simulink model "main_simulator"  (R2021b)
settings: Solver=ode45  StartTime=0.0  StopTime=250  RelTol=1e-3
values from neighbouring files (symbols this model uses):
  a_w = -0.00385    [ParamSetup.m]
  B_r_BP = [0; 0; -1.2]    [ParamSetup.m]    (also in param_set.m = [0; 0; -1.0])
  B_r_BW = [0; 0; 0.1]    [ParamSetup.m]    (also in param_set.m)
  C_BP = eye(3)    [ParamSetup.m]    (also in param_set.m)
  C_BW = eye(3)    [ParamSetup.m]    (also in param_set.m)
  c_Dpd = 3.2    [ParamSetup.m]    (also in param_set.m = 0.5)
  c_Yb = 0.23    [ParamSetup.m]    (also in param_set.m)
  cD = [c_D0; c_Da2; c_Dds]    [ParamSetup.m]    (also in param_set.m = [c_D0; c_DA2; c_DBs; c_DBa])
  cL = [c_L0; c_La; c_Lds]    [ParamSetup.m]    (also in param_set.m = [c_L0; c_LA; c_LBs; c_LBa])
  cM = [c_lp; c_lda; c_m0; c_ma; c_mq; c_nr; c_nda]    [ParamSetup.m]    (also in param_set.m = [c_lp; c_lBa; c_m0; c_mA; c_mq; c_nr; c_nBa])
  F = 0.0555 * (1+8*a_bar^2)*t^2*b^3    [ImIiCompute.m]    (also in param_set.m)
  gravity_acc = + 9.81    (= 9.81)    [ParamSetup.m]    (also in param_set.m)
  heights = linspace(1e-6, 350, wind_pf_size)    [Casadi_guidance.m]    (also in ParamSetup.m = linspace(1e-6, height_lim, wind_pf_size))
  Ii = diag([D, E, F])    [ImIiCompute.m]    (also in param_set.m)
  Im = diag([A, B, C])    [ImIiCompute.m]    (also in param_set.m)
  parafoil_ref_area = 1.5    [ParamSetup.m]    (also in param_set.m)
  parafoil_ref_length = 0.80    (= 0.8)    [ParamSetup.m]    (also in param_set.m)
  parafoil_ref_span = 1.88    [ParamSetup.m]    (also in param_set.m)
  psi_dot_max = 0.2187    [MPC.m]    (also in MPC_2d_path_following_func.m; MPC_2d_path_following_ground_func.m; MPC_3d_path_following.m; MPC_3d_path_following_func.m)
  r = 1000    [MPC.m]
  S_pd = 0.06    [ParamSetup.m]    (also in param_set.m)
  system_mass = 2.2    [ParamSetup.m]    (also in param_set.m)
  wind_profile_hat = GetWindProfile(heights)    [Casadi_guidance.m]    (also in ParamSetup.m)
  xy_dot = 4.59    [MPC.m]    (also in MPC_2d_path_following_func.m; MPC_2d_path_following_ground_func.m; MPC_3d_path_following.m; MPC_3d_path_following_func.m)
  z_dot = 1.39    [MPC.m]    (also in MPC_2d_path_following_func.m; MPC_2d_path_following_ground_func.m; MPC_3d_path_following.m; MPC_3d_path_following_func.m)
undefined symbols (not defined in the file or in its folder): aeroF_est_noise_var, Delta_s, diag_sigma_zeta, Light, MIL, normalize_const, psi_desire, sampling_T, time_horizon_N, wind_est_dyn_var, wind_est_noise_var, xi
libraries: aerolibwind2 x3, simulink x2, sharedtransform x1, shared6dof x1, sensorinslib x1, aerolibatmos2 x1, uavutilslib x1, commchan3 x1, matrix_library x1
settings Model: Creator=zhongyuliang  LastModifiedBy=zhongyuliang

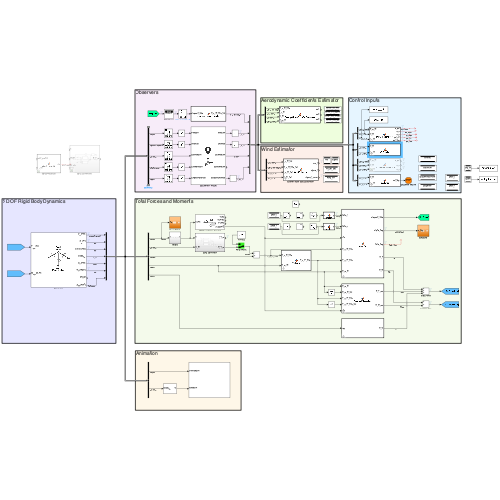
[thumbnail: Simulink's stored preview of the top-level diagram]
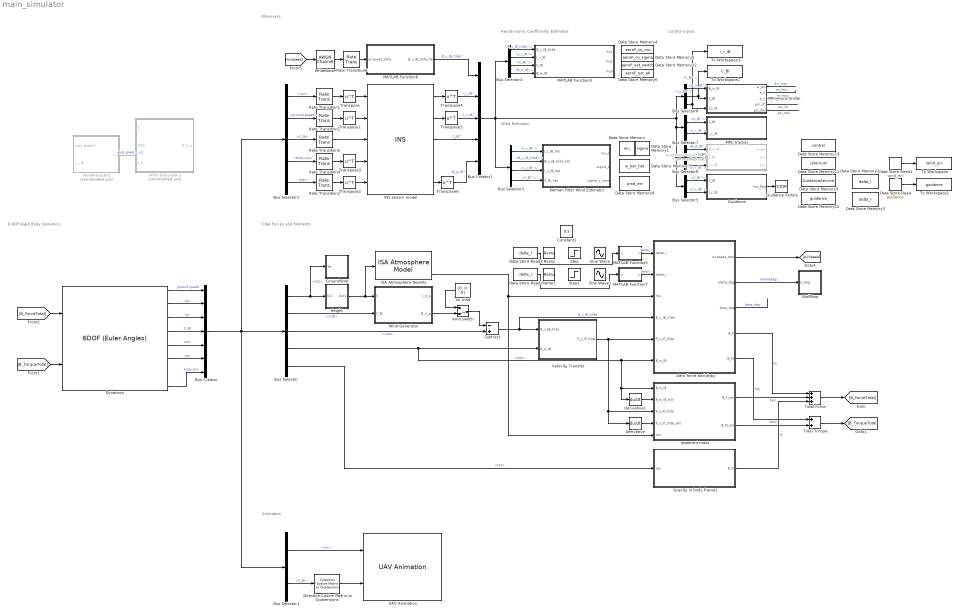
== system main_simulator ==
  note: Total Forces and Moments
  note: Animation
  note: 6 DOF Rigid Body Dynamics
  note: Observers
  note: Wind Estimator
  note: Aerodynamic Coefficients Estimator
  note: Control Inputs
  Aero force and drag : MATLAB Function  TreatAsAtomicUnit=on  mask{cL=cL, cD=cD, cYb=c_Yb, cM=cM, b=parafoil_ref_span, c=parafoil_ref_length, ref_area=parafoil_ref_area, B_r_BP=B_r_BP, C_BP=C_BP, S_pd=S_pd, c_Dpd=c_Dpd, B_r_BW=B_r_BW, C_BW=C_BW}
      mask prompts: cL "lift force coefficients"; cD "drag force coefficients"; cYb "side force coefficients"; cM "moment coefficients"; b "parafoil_ref_span"; c "parafoil_ref_length"; ref_area "parafoil_ref_area"; B_r_BP "origin deviation B_r_BP"; C_BP "rotation matrix C_BP"; S_pd "payload ref area"; c_Dpd "payload drag coefficient"; B_r_BW "origin deviation B_r_BW"; C_BW "rotation matrix C_BW"
  Bus Creator : BusCreator  Inputs=7
  Bus Creator1 : BusCreator  Inputs=5
  Bus Selector : BusSelector  OutputSignals=xyz,C_BI,uvw,pqr,rpy
  Bus Selector1 : BusSelector  OutputSignals=xyz,C_BI
  Bus Selector2 : BusSelector  OutputSignals=xyz,ground speed,C_BI,body acc,pqr
  Bus Selector3 : BusSelector  OutputSignals=I_r_IB^,B_v_IB_tilde^,I_v_IB^,C_BI^
  Bus Selector4 : BusSelector  OutputSignals=B_v_IB_tilde^,I_r_IB^,C_BI^,B_w_IB^
  Bus Selector5 : BusSelector  OutputSignals=C_BI^,I_r_IB^
  Bus Selector6 : BusSelector  OutputSignals=B_w_IB^,C_BI^,I_r_IB^
  Bus Selector7 : BusSelector  OutputSignals=C_BI^,I_r_IB^
  Bus Selector8 : BusSelector  OutputSignals=B_w_IB^,C_BI^,I_r_IB^
  Constant1 : Constant  Value=0.5
  Data Store Memory : DataStoreMemory  DataStoreName=mu  ReadBeforeWriteMsg=warning  WriteAfterWriteMsg=warning  WriteAfterReadMsg=warning  InitialValue=mu0  VectorParams1D=off  ShowAdditionalParam=off  OutDataTypeStr=double
  Data Store Memory1 : DataStoreMemory  DataStoreName=sigma  ReadBeforeWriteMsg=warning  WriteAfterWriteMsg=warning  WriteAfterReadMsg=warning  InitialValue=sigma0  VectorParams1D=off  ShowAdditionalParam=off  OutDataTypeStr=double
  Data Store Memory10 : DataStoreMemory  DataStoreName=guidance  ReadBeforeWriteMsg=warning  WriteAfterWriteMsg=warning  WriteAfterReadMsg=warning  InitialValue=zeros(4,2000)  ShowAdditionalParam=off  OutDataTypeStr=double
  Data Store Memory11 : DataStoreMemory  DataStoreName=colornum  ReadBeforeWriteMsg=warning  WriteAfterWriteMsg=warning  WriteAfterReadMsg=warning  InitialValue=randi([1,11],1)  ShowAdditionalParam=off  OutDataTypeStr=double
  Data Store Memory12 : DataStoreMemory  DataStoreName=aeroF_est_switch  ReadBeforeWriteMsg=warning  WriteAfterWriteMsg=warning  WriteAfterReadMsg=warning  InitialValue=[0,0]  VectorParams1D=off  ShowAdditionalParam=off  OutDataTypeStr=double
  Data Store Memory13 : DataStoreMemory  DataStoreName=control  ReadBeforeWriteMsg=warning  WriteAfterWriteMsg=warning  WriteAfterReadMsg=warning  InitialValue=control0  ShowAdditionalParam=off  OutDataTypeStr=double
  Data Store Memory2 : DataStoreMemory  DataStoreName=delta_l  ReadBeforeWriteMsg=warning  WriteAfterWriteMsg=warning  WriteAfterReadMsg=warning  InitialValue=0.5  ShowAdditionalParam=off  OutDataTypeStr=double
  Data Store Memory3 : DataStoreMemory  DataStoreName=delta_r  ReadBeforeWriteMsg=warning  WriteAfterWriteMsg=warning  WriteAfterReadMsg=warning  InitialValue=0.5  ShowAdditionalParam=off  OutDataTypeStr=double
  Data Store Memory4 : DataStoreMemory  DataStoreName=aeroF_co_mu  ReadBeforeWriteMsg=warning  WriteAfterWriteMsg=warning  WriteAfterReadMsg=warning  InitialValue=aeroF_co_mu0  VectorParams1D=off  ShowAdditionalParam=off  OutDataTypeStr=double
  Data Store Memory5 : DataStoreMemory  DataStoreName=aeroF_co_sigma  ReadBeforeWriteMsg=warning  WriteAfterWriteMsg=warning  WriteAfterReadMsg=warning  InitialValue=aeroF_co_sigma0  VectorParams1D=off  ShowAdditionalParam=off  OutDataTypeStr=double
  Data Store Memory6 : DataStoreMemory  DataStoreName=aeroF_est_ab  ReadBeforeWriteMsg=warning  WriteAfterWriteMsg=warning  WriteAfterReadMsg=warning  InitialValue=[0, 0, 0; 0, 0, 0]  VectorParams1D=off  ShowAdditionalParam=off  OutDataTypeStr=double
  Data Store Memory7 : DataStoreMemory  DataStoreName=w_bar_hat  ReadBeforeWriteMsg=warning  WriteAfterWriteMsg=warning  WriteAfterReadMsg=warning  InitialValue=w_bar_hat0  VectorParams1D=off  ShowAdditionalParam=off  OutDataTypeStr=double
  Data Store Memory8 : DataStoreMemory  DataStoreName=wind_err  ReadBeforeWriteMsg=warning  WriteAfterWriteMsg=warning  WriteAfterReadMsg=warning  InitialValue=wind_err0  VectorParams1D=off  ShowAdditionalParam=off  OutDataTypeStr=double
  Data Store Memory9 : DataStoreMemory  DataStoreName=GuidanceService  ReadBeforeWriteMsg=warning  WriteAfterWriteMsg=warning  WriteAfterReadMsg=warning  InitialValue=1  ShowAdditionalParam=off  OutDataTypeStr=double
  Data Store Read : DataStoreRead  DataStoreName=guidance  IndexOptions=Index vector (dialog)  Indices=1  OutputSizes=1
  Data Store Read1 : DataStoreRead  DataStoreName=wind_err  IndexOptions=Index vector (dialog)  Indices=1  OutputSizes=1
  Data Store Read2 : DataStoreRead  DataStoreName=delta_l  IndexOptions=Index vector (dialog)  Indices=1  OutputSizes=1
  Data Store Read3 : DataStoreRead  DataStoreName=delta_r  IndexOptions=Index vector (dialog)  Indices=1  OutputSizes=1
  Derivative : Derivative
  Derivative1 : Derivative
  Direction Cosine Matrix to Quaternions : sharedtransform/Direction Cosine Matrix  to Quaternions  aMode=0  action=None  tolerance=eps(2)
      settings: SourceProductBaseCode=AE,PW,DR,MT,UV,VE
  Dynamics : shared6dof/6DOF (Euler Angles)  units=Metric (MKS)  mtype=Fixed  rep=Euler Angles  xme_0=init_pos_in_inertial_frame  Vm_0=init_uvw  eul_0=init_rpy  pm_0=init_pqr  mass_0=system_mass  mass_e=0.5  mass_f=2.0  inertia=system_inertia  inertia_e=eye(3)  inertia_f=2*eye(3)  k_quat=1.0  vre_flag=on  abi_flag=off  aMode=0  xme_statename=''  Vm_statename=''  eul_statename=''  quat_statename=''  pm_statename=''  mass_statename=''
      settings: SourceProductBaseCode=AE,PW,DR,MT,UV,VE
  Gravity in body frame1 : MATLAB Function  ClipboardFcn="m = load(\"params.mat\",\"system_mass\")"  TreatAsAtomicUnit=on  mask{m=system_mass, g=gravity_acc}
      mask prompts: m "system_mass"; g "gravity_acc"
  GroundStop : Subsystem
  Guidance : MATLAB Function  TreatAsAtomicUnit=on  SystemSampleTime=25  mask{heights=heights, Delta_s=Delta_s, z_dot=z_dot, xy_dot=xy_dot, psi_dot_max=psi_dot_max, psi_d=psi_desire}
      mask prompts: Delta_s "wind pos deviation"; z_dot "descending rate no wind"; xy_dot "horizontal vel no wind"; psi_dot_max "max turning rate no wind"; psi_d "desired landing pose"
  Guidance Failure : Stop
  GuidancePDcontroller : MATLAB Function  Commented=on  TreatAsAtomicUnit=on
  Height : Subsystem
  INS sensor model : sensorinslib/INS  MountingLocation=[0 0 0]  RollAccuracy=row_pitch_accu  PitchAccuracy=row_pitch_accu  YawAccuracy=yaw_accu  PositionAccuracy=pos_accu  VelocityAccuracy=vel_accu  UseAccelAndAngVel=on  AccelerationAccuracy=acc_accu  AngularVelocityAccuracy=angVel_accu  TimeInput=off  PositionErrorFactor=[0 0 0]  SeedDouble=67  SimulateUsing=Interpreted execution
      settings: SourceProductBaseCode=DR,TF,NV,UV
  ISA Atmosphere Density : aerolibatmos2/ISA Atmosphere Model  custom=off  g=9.80665  gamma=1.4  R=287.0531  L=0.0065  h_trop=11000  h_strat=20000  rho0=1.225  P0=101325  T0=288.15  h0=0
  Kalman Filter Wind Estimator : MATLAB Function  TreatAsAtomicUnit=on  mask{Q=wind_est_dyn_var, R=wind_est_noise_var, heights=heights, wind_profile_hat=wind_profile_hat, C=normalize_const}
      mask prompts: Q "wind_est_dyn_var"; R "wind_est_noise_var"; wind_profile_hat "forcast wind profile"; C "normalize_const"
  MATLAB Function3 : MATLAB Function  TreatAsAtomicUnit=on  mask{m=system_mass, g=gravity_acc, C_BP=C_BP, C_BW=C_BW, ref_area=parafoil_ref_area, S_pd=S_pd, R=aeroF_est_noise_var}
      mask prompts: m "system_mass"; g "gravity_acc"; C_BP "rotation matrix C_BP"; C_BW "rotation matrix C_BW"; ref_area "parafoil_ref_area"; S_pd "payload_ref_area"; R "aeroF_est_noise_var"
  MATLAB Function5 : MATLAB Function  TreatAsAtomicUnit=on
  MATLAB Function6 : MATLAB Function  TreatAsAtomicUnit=on
  MATLAB Function7 : MATLAB Function  TreatAsAtomicUnit=on
  MPC tracker : MATLAB Function  TreatAsAtomicUnit=on  SystemSampleTime=2.38  mask{xy_dot=xy_dot, z_dot=z_dot, psi_dot_max=psi_dot_max, N=time_horizon_N}
      mask prompts: N "MPC time horizon"
  MPC_PDcontroller : MATLAB Function  TreatAsAtomicUnit=on
  Ramp : simulink/Sources/Ramp  slope=0.03  start=10  InitialOutput=0.5
  Ramp1 : simulink/Sources/Ramp  slope=-0.03  start=10  InitialOutput=0.5
  Rate Transition{1..6} (6 alike) : RateTransition  OutPortSampleTime=sampling_T
  Sine Wave : Sin  Amplitude=0.5  Bias=0.5  SampleTime=0
  Sine Wave1 : Sin  Amplitude=0.5  Bias=0.5  SampleTime=0
  StallStop : Subsystem
  Step : Step  Time=20  SampleTime=0
  Step1 : Step  Time=20  SampleTime=0
  Subtract : Sum  Inputs=-+
  To Workspace : ToWorkspace  VariableName=wind_err  SaveFormat=Structure With Time  SampleTime=-1
  To Workspace1 : ToWorkspace  VariableName=guidance  SaveFormat=Structure With Time  SampleTime=-1
  To Workspace2 : ToWorkspace  VariableName=C_BI  SaveFormat=Structure With Time  SampleTime=-1
  To Workspace3 : ToWorkspace  VariableName=I_r_IB  SaveFormat=Structure With Time  SampleTime=-1
  Total Force : Sum  Inputs=+++
  Total Torque : Sum
  Transpose{,1..6} (7 alike) : Math  Operator=transpose  SaturateOnIntegerOverflow=on
  UAV Animation : uavutilslib/UAV Animation  UAVType=FixedWing  UAVSize=40  InertialZDirection=Down  SampleTime=-1
      settings: SourceProductBaseCode=UV
  Velovity Transfer : MATLAB Function  TreatAsAtomicUnit=on  mask{B_r_BP=B_r_BP, C_BP=C_BP}
  WhiteNoise : commchan3/AWGN Channel  InputProcessing=Columns as channels (frame based)  seed=67  noiseMode=Variance from mask  EbNodB=10  EsNodB=10  SNRdB=100  bitsPerSym=1  Ps=1  Tsym=1  variance=airspeed_var
  Wind Generator : Subsystem
  Wind Generator1 : Subsystem  Commented=on
  WindPredictViz : MATLAB Function  Commented=on  TreatAsAtomicUnit=on  SystemSampleTime=sampling_T
  apparent mass : MATLAB Function  TreatAsAtomicUnit=on  mask{Im=Im, Ii=Ii, B_r_BP=B_r_BP, C_BP=C_BP}
      mask prompts: Im "apparent mass / air density"; Ii "apparent inertia / air density"; B_r_BP "origin deviation B_r_BP"; C_BP "rotation matrix C_BP"
  no wind : Constant  Value=[0; 0; 0]
  wind switch : ManualSwitch  CurrentSetting=0
  wires:
  Bus Selector/3 -> Subtract/2  "<uvw>"
  Height/1(Out1) -> Wind Generator/1(h), ISA Atmosphere Density/1
  Subtract/1 -> Velovity Transfer/1(B_v_IB_tilde), Aero force and drag/4(B_v_IB_tilde)  "B_v_IB_tilde"
  Velovity Transfer/1(P_v_IP_tilde) -> Aero force and drag/5(P_v_IP_tilde), apparent mass/3(P_v_IP_tilde), Derivative/1
  ISA Atmosphere Density/4 -> apparent mass/5(rho), Aero force and drag/3(rho)
  Derivative/1 -> apparent mass/4(P_v_IP_tilde_dot)
  Bus Selector/5 -> Gravity in body frame1/1(rpy)  "<rpy>"
  [B_ForceTotal] -> Dynamics/1
  [B_TorqueTotal] -> Dynamics/2
  Derivative1/1 -> apparent mass/2(B_w_IB_dot)
  Bus Selector/1 -> Height/1(In1), GroundStop/1(Xe)  "<xyz>"
  Direction Cosine Matrix to Quaternions/1 -> UAV Animation/2
  Bus Selector/4 -> Velovity Transfer/2(B_w_IB), Aero force and drag/6(B_w_IB), apparent mass/1(B_w_IB), Derivative1/1  "<pqr>"
  Dynamics/1 -> Bus Creator/1  "ground speed"
  Dynamics/2 -> Bus Creator/2  "xyz"
  Dynamics/3 -> Bus Creator/3  "rpy"
  Dynamics/4 -> Bus Creator/4  "C_BI"
  Dynamics/5 -> Bus Creator/5  "uvw"
  Dynamics/6 -> Bus Creator/6  "pqr"
  Dynamics/8 -> Bus Creator/7  "body acc"
  Bus Creator/1 -> Bus Selector/1, Bus Selector1/1, Bus Selector2/1
  Bus Selector1/1 -> UAV Animation/1  "<xyz>"
  Bus Selector1/2 -> Direction Cosine Matrix to Quaternions/1  "<C_BI>"
  Bus Selector/2 -> Wind Generator/2(C_BI)  "<C_BI>"
  MATLAB Function5/1(y) -> Aero force and drag/1(delta_l)  "delta_l"
  MATLAB Function7/1(y) -> Aero force and drag/2(delta_r)  "delta_r"
  no wind/1 -> wind switch/1
  Wind Generator/2(B_V_w) -> wind switch/2
  wind switch/1 -> Subtract/1
  Aero force and drag/1(airspeed_data) -> [AirSpeed]
  Aero force and drag/5(B_M) -> Total Torque/1  "Ma"
  Gravity in body frame1/1(B_G) -> Total Force/3  "G"
  Total Torque/1 -> [B_TorqueTotal]
  Total Force/1 -> [B_ForceTotal]
  Aero force and drag/4(B_F) -> Total Force/1  "Fa"
  apparent mass/2(B_M_am) -> Total Torque/2  "Mam"
  Aero force and drag/2(alpha_deg) -> StallStop/1(a_deg)  "alpha[deg]"
  Bus Selector2/4 -> Rate Transition4/1  "<body acc>"
  Bus Selector3/2 -> Kalman Filter Wind Estimator/2(B_v_IB_tilde_hat)  "<B_v_IB_tilde^>"
  Bus Selector3/1 -> Kalman Filter Wind Estimator/1(I_r_IB_hat)  "<I_r_IB^>"
  Rate Transition2/1 -> Transpose1/1
  MATLAB Function6/1(B_v_IB_tilde_hat) -> Bus Creator1/1  "B_v_IB_tilde^"
  Bus Selector4/4 -> MATLAB Function3/4(B_w_IB)  "<B_w_IB^>"
  Bus Selector3/4 -> Kalman Filter Wind Estimator/4(C_BI_hat)  "<C_BI^>"
  Bus Selector6/1 -> GuidancePDcontroller/1(B_w_IB)  "<B_w_IB^>"
  WhiteNoise/1 -> Rate Transition6/1
  INS sensor model/3 -> Bus Creator1/4  "C_BI^"
  Bus Selector5/1 -> Guidance/1(C_BI)  "<C_BI^>"
  Transpose/1 -> INS sensor model/1
  Rate Transition1/1 -> Transpose/1
  Rate Transition3/1 -> Transpose2/1
  Transpose3/1 -> INS sensor model/4
  [AirSpeed] -> WhiteNoise/1
  Bus Selector3/3 -> Kalman Filter Wind Estimator/3(I_v_IB_hat)  "<I_v_IB^>"
  Transpose5/1 -> Bus Creator1/3  "I_v_IB^"
  Rate Transition6/1 -> MATLAB Function6/1(airspeed_data)
  INS sensor model/5 -> Transpose6/1
  INS sensor model/1 -> Transpose4/1
  Rate Transition5/1 -> INS sensor model/3
  Bus Selector2/3 -> Rate Transition5/1  "<C_BI>"
  Guidance/1(not_flag) -> Guidance Failure/1
  Transpose2/1 -> INS sensor model/5
  Bus Selector2/1 -> Rate Transition1/1  "<xyz>"
  Bus Selector2/2 -> Rate Transition2/1  "<ground speed>"
  Bus Selector2/5 -> Rate Transition3/1  "<pqr>"
  Transpose1/1 -> INS sensor model/2
  INS sensor model/2 -> Transpose5/1
  Bus Selector6/3 -> GuidancePDcontroller/3(I_r_IB)  "<I_r_IB^>"
  Transpose6/1 -> Bus Creator1/5  "B_w_IB^"
  Bus Selector6/2 -> GuidancePDcontroller/2(C_BI)  "<C_BI^>"
  Transpose4/1 -> Bus Creator1/2  "I_r_IB^"
  Bus Selector5/2 -> Guidance/2(I_r_IB)  "<I_r_IB^>"
  Rate Transition4/1 -> Transpose3/1
  Bus Selector4/2 -> MATLAB Function3/2(I_r_IB)  "<I_r_IB^>"
  Bus Selector4/1 -> MATLAB Function3/1(B_v_IB_tilde)  "<B_v_IB_tilde^>"
  Bus Selector4/3 -> MATLAB Function3/3(C_BI)  "<C_BI^>"
  WindPredictViz/1(viz) -> ?  "wind_predict_viz"
  apparent mass/1(B_F_am) -> Total Force/2  "Fam"
  Aero force and drag/3(beta_deg) -> ?  "beta_deg"
  Data Store Read2/1 -> MATLAB Function5/1(u)
  Data Store Read3/1 -> MATLAB Function7/1(u)
  Data Store Read/1 -> To Workspace1/1
  Data Store Read1/1 -> To Workspace/1
  Bus Selector7/1 -> MPC tracker/1(C_BI)  "<C_BI^>"
  Bus Selector7/2 -> MPC tracker/2(I_r_IB)  "<I_r_IB^>"
  Bus Creator1/1 -> Bus Selector4/1, Bus Selector3/1, Bus Selector8/1, Bus Selector5/1, Bus Selector6/1, Bus Selector7/1
  Bus Selector8/1 -> MPC_PDcontroller/1(B_w_IB)  "<B_w_IB^>"
  Bus Selector8/2 -> To Workspace2/1, MPC_PDcontroller/2(C_BI)  "<C_BI^>"
  MPC_PDcontroller/1(e_psi) -> ?  "err_mpc"
  Bus Selector8/3 -> To Workspace3/1, MPC_PDcontroller/3(I_r_IB)  "<I_r_IB^>"
  MPC_PDcontroller/2(e_x) -> ?  "ex_mpc"
  MPC_PDcontroller/3(e_y) -> ?  "ey_mpc"
  MPC_PDcontroller/4(psi_ctl) -> ?  "psi_ctl"
  MPC_PDcontroller/5(psi_des) -> ?  "psi_des"

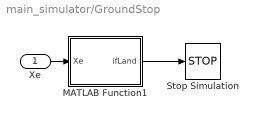
== system main_simulator/GroundStop ==
  Xe : Inport
  MATLAB Function1 : MATLAB Function  TreatAsAtomicUnit=on
  Stop Simulation : Stop
  wires:
  Xe/1 -> MATLAB Function1/1(Xe)
  MATLAB Function1/1(ifLand) -> Stop Simulation/1

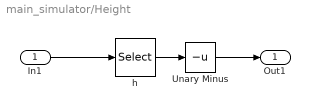
== system main_simulator/Height ==
  In1 : Inport
  Unary Minus : UnaryMinus
  h : Selector  InputPortWidth=3  IndexOptions=Index vector (dialog)  Indices=3  OutputSizes=1
  Out1 : Outport
  wires:
  Unary Minus/1 -> Out1/1
  In1/1 -> h/1
  h/1 -> Unary Minus/1

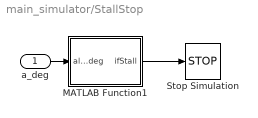
== system main_simulator/StallStop ==
  a_deg : Inport
  MATLAB Function1 : MATLAB Function  TreatAsAtomicUnit=on
  Stop Simulation : Stop
  wires:
  a_deg/1 -> MATLAB Function1/1(alpha_deg)
  MATLAB Function1/1(ifStall) -> Stop Simulation/1

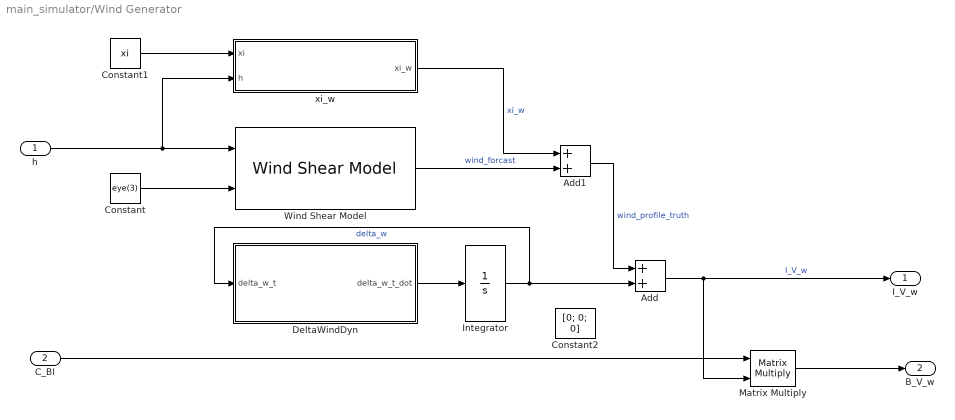
== system main_simulator/Wind Generator ==
  h : Inport
  C_BI : Inport  Port=2
  Add : Sum
  Add1 : Sum
  Constant : Constant  Value=eye(3)
  Constant1 : Constant  Value=xi
  Constant2 : Constant  Value=[0; 0; 0]
  DeltaWindDyn : MATLAB Function  TreatAsAtomicUnit=on  SystemSampleTime=0.2  mask{a_w=a_w, diag_sigma_zeta=diag_sigma_zeta}
  Integrator : Integrator
  Matrix Multiply : Product  Multiplication=Matrix(*)
  Wind Shear Model : aerolibwind2/Wind Shear Model  units=Metric (MKS)  phase=Category C - Terminal Flight Phase  W_20=vel_at6m  Wdeg=theta
  xi_w : MATLAB Function  TreatAsAtomicUnit=on
  I_V_w : Outport
  B_V_w : Outport  Port=2
  wires:
  DeltaWindDyn/1(delta_w_t_dot) -> Integrator/1
  Wind Shear Model/1 -> Add1/2  "wind_forcast"
  Add/1 -> I_V_w/1, Matrix Multiply/2  "I_V_w"
  h/1 -> xi_w/2(h), Wind Shear Model/1
  Integrator/1 -> Add/2, DeltaWindDyn/1(delta_w_t)  "delta_w"
  C_BI/1 -> Matrix Multiply/1
  Matrix Multiply/1 -> B_V_w/1
  Constant/1 -> Wind Shear Model/2
  Constant1/1 -> xi_w/1(xi)
  xi_w/1(xi_w) -> Add1/1  "xi_w"
  Add1/1 -> Add/1  "wind_profile_truth"

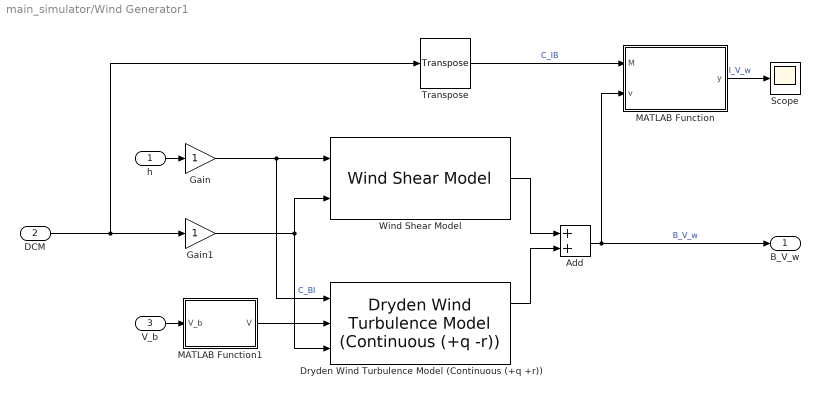
== system main_simulator/Wind Generator1 ==
  h : Inport
  DCM : Inport  Port=2
  V_b : Inport  Port=3
  Add : Sum
  Dryden Wind Turbulence Model (Continuous (+q +r)) : aerolibwind2/Dryden Wind Turbulence Model  (Continuous (+q -r))  units=Metric (MKS)  spec=MIL-F-8785C  model=Continuous Dryden (+q +r)  W20=turbulence_vel_at6m  Wdeg=turbulence_ori_at6m  TurbProb=10^-2 - Light  L_high=533.4  Wingspan=parafoil_ref_span  ts=0.1  Seed=[23341 23342 23343 23344]  T_on=on
  Gain : Gain
  Gain1 : Gain
  MATLAB Function : MATLAB Function  TreatAsAtomicUnit=on
  MATLAB Function1 : MATLAB Function  TreatAsAtomicUnit=on
  Scope : Scope
  Transpose : matrix_library/Transpose
      settings: SourceProductBaseCode=SL
  Wind Shear Model : aerolibwind2/Wind Shear Model  units=Metric (MKS)  phase=Category C - Terminal Flight Phase  W_20=laminar_wind_vel_at6m  Wdeg=laminar_wind_ori_at6m
  B_V_w : Outport
  wires:
  V_b/1 -> MATLAB Function1/1(V_b)
  DCM/1 -> Transpose/1, Gain1/1
  Dryden Wind Turbulence Model (Continuous (+q +r))/1 -> Add/2
  MATLAB Function1/1(V) -> Dryden Wind Turbulence Model (Continuous (+q +r))/2
  h/1 -> Gain/1
  Gain/1 -> Dryden Wind Turbulence Model (Continuous (+q +r))/1, Wind Shear Model/1
  Wind Shear Model/1 -> Add/1
  Gain1/1 -> Dryden Wind Turbulence Model (Continuous (+q +r))/3, Wind Shear Model/2  "C_BI"
  Add/1 -> B_V_w/1, MATLAB Function/2(v)  "B_V_w"
  MATLAB Function/1(y) -> Scope/1  "I_V_w"
  Transpose/1 -> MATLAB Function/1(M)  "C_IB"

== matlab function main_simulator/Gravity in body frame1 ==
  data: rpy input; B_G output; m parameter; g parameter
function B_G = GravityInBodyFrame(rpy, m, g)
    B_G = m*g*[-sin(rpy(2));
             sin(rpy(1))*cos(rpy(2));
             cos(rpy(1))*cos(rpy(2))];
end

== matlab function main_simulator/GroundStop/MATLAB Function1 ==
  data: Xe input; ifLand output
function ifLand = logic(Xe)

    if Xe(3) < -0.000001
        ifLand = 0;
    else
        ifLand = 1;
    end

end

== matlab function main_simulator/StallStop/MATLAB Function1 ==
  data: alpha_deg input; ifStall output
function ifStall = logic(alpha_deg)

    if alpha_deg < 45
        ifStall = 0;
    else
        ifStall = 1;
    end
%     ifStall = 0;

end

== matlab function main_simulator/Wind Generator/xi_w ==
  data: xi input; h input; xi_w output
function xi_w = fcn(xi,h)

xi_w = [xi(1) * h / 200;
        xi(2) * h / 200;
        0];
end

== matlab function main_simulator/Guidance ==
  settings: updateMethod=DISCRETE
  data: not_flag output; C_BI input; I_r_IB input; heights parameter; psi_dot_max parameter; xy_dot parameter; z_dot parameter; psi_d parameter; Delta_s parameter; guidance data_store_memory; GuidanceService data_store_memory
function not_flag = Guidance(C_BI, I_r_IB, heights, psi_dot_max, xy_dot, z_dot, psi_d, Delta_s)

    global GuidanceService;
    global guidance
    h = -I_r_IB(3);
    not_flag = false;

    
    if h<300 && h>1e-6 && GuidanceService
        disp('------Guidance------')
        Vz = z_dot;
        Dx_w = (1/Vz)*interp1(heights, Delta_s(1,:), h, 'linear','extrap');
        Dy_w = (1/Vz)*interp1(heights, Delta_s(2,:), h, 'linear','extrap');
        V0 = xy_dot / Vz;
        T = h;
        um = psi_dot_max / Vz;

        C_IB = C_BI';
        psi0 = atan2(C_IB(2,1), C_IB(1,1));
        
        init_pose = [I_r_IB(1) + Dx_w;
                     I_r_IB(2) + Dy_w;
                     psi0];
        final_pose = [0; 0; psi_d];
        
        % NLP solver
        [p_0_star, ~, flag] = fminsearch(@(P0) ComputeErr(P0, init_pose, final_pose, T, V0, um),[-1e-5,1e-5,1e-4],optimset('TolFun',1e-7,'TolX',1e-7,'MaxFunEvals',1e5,'MaxIter',1e5));
        not_flag = ~flag;
        
        % if solution found
        if flag
            t_span = linspace(0, T, 2000);
            x0 = [init_pose(1);
                  init_pose(2);
                  init_pose(3);
                  p_0_star(1);
                  p_0_star(2);
                  p_0_star(3)];
            [time, traj] = ode45(@(t,x) ODEdyn(t,x, V0, um), t_span, x0);
        
            for i = 1:2000
                guidance(:,i) = [traj(i,1) - (1/Vz)*interp1(heights, Delta_s(1,:), h - time(i),'linear','extrap'); % I_rx
                                 traj(i,2) - (1/Vz)*interp1(heights, Delta_s(2,:), h - time(i),'linear','extrap'); % I_ry
                                 h - time(i); % h, -I_rz
                                 traj(i,3)]; % psi
            end
            
            % plot
            hold on
            grid on
            xlabel('East --> y') 
            ylabel('North --> x') 
            zlabel('Height --> h')
            plot3(guidance(2,:),guidance(1,:),guidance(3,:),'k') % changed viz axis
            
        else
            disp("Warning! Guidance solver failed!")
            return % guidance fail! do not update guidance, go to teleop...
        end
        GuidanceService = 0; % task complete
    end
end

function dxdt = ODEdyn(t, x, V0, um) % x = [x, y, chi, p1, p2, p3]^T
    if(x(6) >= 2*um)
        u = -um;
    elseif(x(6) >= -2*um)
        u = -x(6)/2;
    else
        u = um;
    end
    dxdt = [V0*cos(x(3));
            V0*sin(x(3));
            u;
            0;
            0;
            x(4)*V0*sin(x(3)) - x(5)*V0*cos(x(3))];
end

function err = ComputeErr(P0, init_pose, final_pose, T, V0, um)
    t_span = linspace(0, T, 1000);
    x0 = [init_pose(1);
          init_pose(2);
          init_pose(3);
          P0(1);
          P0(2);
          P0(3)];
    [~, traj] = ode45(@(t,x) ODEdyn(t,x, V0, um), t_span, x0);
    err = sqrt((traj(end,1) - final_pose(1))^2 + (traj(end,2) - final_pose(2))^2) - 10000*((cos(traj(end,3) - final_pose(3)) -1));
end

== matlab function main_simulator/MPC tracker ==
  data: C_BI input; I_r_IB input; guidance data_store_memory; wind_err data_store_memory; z_dot parameter; xy_dot parameter; control data_store_memory; psi_dot_max parameter; N parameter; GuidanceService data_store_memory
function MPCtracker(C_BI, I_r_IB, z_dot, xy_dot, psi_dot_max, N)
    coder.extrinsic("MPC_func")

    global guidance
    global wind_err
    global control
    global GuidanceService

    % get current state
    xc = I_r_IB(1);
    yc = I_r_IB(2);
    h = -I_r_IB(3);
    C_IB = C_BI';
    psi_c = atan2(C_IB(2,1), C_IB(1,1));

    if isnan(xc) || isnan(yc) || isnan(h) || isnan(psi_c)
        disp("Warning: MPCtracker early return because of NaN current pose value")
        return
    elseif h < 1e-6
        disp("Warning: MPCtracker early return because h < 1e-6")
        return
    end

    % if guidance and wind_err received
    zero_cnt = sum(guidance==0, 'all') + sum(wind_err==0, 'all');

    if zero_cnt<3

        [~, id] = min(abs(guidance(3,:) - h*ones(1,2000)));
        x0 = guidance(1,id);
        y0 = guidance(2,id);
        dx = mean(wind_err(2,:));
        dy = mean(wind_err(3,:));
        dh = (guidance(3,1) - guidance(3,end))/(2000 - 1);
        Ts = dh / z_dot;
        init_pose = [xc - x0; yc - y0; psi_c];
        
        % Compute ref trajectory
        ref = zeros(3,N);
        ref(3,1) = guidance(4,id);
        for i = 2:N
            if id+i-1>2000
                ref(:,i) = ref(:,i-1);
            else
                ref(:,i) =  [ref(1,i-1) + Ts * xy_dot * cos(guidance(4,id+i-2));
                             ref(2,i-1) + Ts * xy_dot * sin(guidance(4,id+i-2));
                             guidance(4,id+i-1)];
            end
        end
        
        % Solve MPC problem
        flag = true;
        xs = zeros(3,N); % define output shape
        us = zeros(1,N-1); % define output shape
        P = diag([10000,10000,100]);
        Q = diag([100, 100, 10000]);
        Qn = diag([1000, 1000, 100]);
        r = 1000;
        um = psi_dot_max;
        
        if sum(isnan(init_pose),'all')>0
            disp("Warning: MPCtracker early return because of NaN initial pose value")
        elseif sum(isnan(ref),'all')>0
            disp("Warning: MPCtracker early return because of NaN reference value")
        end

        [flag, xs, ~] = MPC_func(N, init_pose, P, Q, r, Qn, ref, Ts, xy_dot, um, dx, dy);
        if flag
            if id+N-1 <= 2000
                ctl = [guidance(3,id:id+N-1);
                       xs(3,:)];
                control = ctl(:,1:size(control,2));
            else
                ctl = [guidance(3,id:2000), linspace(-dh, -dh*(N-(2000-id+1)), N-(2000-id+1));
                       xs(3,:)];
                control = ctl(:,1:size(control,2));
            end        
        else
            disp("MPC solver failed")
            GuidanceService = 1; % recall guidance, do not change control in buffer
        end
    end
end

== matlab function main_simulator/MATLAB Function5 ==
  data: u input; y output
function y = motor(u)
    if u>1
        y = 1;
    elseif u<0
        y = 0;
    else
        y = u;
    end
end

== matlab function main_simulator/MPC_PDcontroller ==
  data: B_w_IB input; C_BI input; I_r_IB input; delta_l data_store_memory; delta_r data_store_memory; guidance data_store_memory; control data_store_memory; GuidanceService data_store_memory; colornum data_store_memory; e_psi output; e_x output; e_y output; psi_ctl output; psi_des output
function [e_psi, e_x, e_y, psi_ctl, psi_des] = MPC_PDcontroller(B_w_IB, C_BI, I_r_IB)
    global delta_l
    global delta_r
    global control
    global GuidanceService
    global guidance
    global colornum
    
    % get current state
    h = -I_r_IB(3);
    C_IB = C_BI';
    x_now = I_r_IB(1);
    y_now = I_r_IB(2);
    psi_now = atan2(C_IB(2,1), C_IB(1,1));

    % plot current state
    hold on;
    colorcode = {"g","b", "c", "m", "#0072BD", "#D95319", "#EDB120", "#7E2F8E", "#77AC30", "#4DBEEE", "#A2142F"};
    states_now = [y_now,                x_now,                h;
                  y_now+1*sin(psi_now), x_now+1*cos(psi_now), h];
    plot3(states_now(:,1), states_now(:,2), states_now(:,3), 'color', colorcode{colornum});

    % default output
    e_psi = 0;
    e_x = 0;
    e_y = 0;
    psi_ctl = 0; % for debug
    psi_des = 0; % for debug
    
    if isnan(x_now) || isnan(y_now) || isnan(h) || isnan(psi_now)
        disp("Warning: MPC_PDcontroller early return because of NaN value")
        return
%     elseif h < 1e-6
%         disp("Warning: GuidancePDcontroller early return because h < 1e-6")
%         return
    end

    % get control
    zero_cnt = sum(control==0, 'all') + sum(guidance==0, 'all'); % if control and guidance received
    if zero_cnt<3
        x_des = interp1(guidance(3,:), guidance(1,:), h, 'linear','extrap'); 
        y_des = interp1(guidance(3,:), guidance(2,:), h, 'linear','extrap'); 
        psi_des = interp1(guidance(3,:), guidance(4,:), h, 'linear','extrap'); 
       
        % plot desired trajectory
        traj = [y_des,                x_des,                h;
                y_des+1*sin(psi_des), x_des+1*cos(psi_des), h];
        plot3(traj(:,1), traj(:,2), traj(:,3), 'r');

        e1 = x_now - x_des;
        e2 = y_now - y_des;
        e_x = e1*cos(psi_des) + e2*sin(psi_des);
        e_y = - e1*sin(psi_des) + e2*cos(psi_des);

        
%         if h<50 && (e_x>10 || e_x<-10 || abs(e_y)>10)
%             GuidanceService = 1; % call guidance service again
%             return
%         end

        % PD control
        psi_dot_now = B_w_IB(3); % approximately
        psi_ctl = interp1(control(1,:), control(2,:), h, 'linear', 'extrap');

        kp = 3; % kp >= 0
        kd = 0.1; % kd >= 0
        kpx = 0.5; % kpx >= 0

        e_psi = warpToPi(psi_now - psi_ctl); % in [-pi, pi]
        u = kp * e_psi + kd * psi_dot_now;
%         ux = kpx * e_x; % compensate x deviation
%             
%         % heuristic allocation
%         u = max(min(u, 0.5),-0.5); % track psi first
%         if u > 0
%             ux = max(min(ux, 0.5-u), u-0.5); % change delta_s to control velocity
%         else
%             ux = max(min(ux, 0.5+u), -u-0.5);
%         end

        delta_l = 0.5 + u ; % if u>0, turn left
        delta_r = 0.5 - u ; % if ux>0, slow down
    end
end

function alpha = warpToPi(theta)
    theta = mod(theta, 2*pi);
    if theta > pi
        alpha = theta - 2*pi;
    else
        alpha = theta;
    end
end

== matlab function main_simulator/Wind Generator1/MATLAB Function ==
  data: M input; y output; v input
function y = MatrixMultiVec(M,v)

    y = M*v;
end

== matlab function main_simulator/MATLAB Function6 ==
  data: airspeed_data input; B_v_IB_tilde_hat output
function B_v_IB_tilde_hat = airspeed_sensor_model(airspeed_data)
    alpha = airspeed_data(1);
    beta = airspeed_data(2);
    Vb = airspeed_data(3);
    B_v_IB_tilde_hat = Vb*[cot(alpha)*abs(sin(alpha)*cos(beta));
                           sin(beta);
                           abs(sin(alpha)*cos(beta)) ];
end

== matlab function main_simulator/Kalman Filter Wind Estimator ==
  data: I_r_IB_hat input; B_v_IB_tilde_hat input; I_v_IB_hat input; C_BI_hat input; mu_t output; sigma_t output; mu data_store_memory; sigma data_store_memory; R parameter; sigma_t_norm output; Q parameter; w_bar_hat data_store_memory; heights parameter; wind_profile_hat parameter; wind_err data_store_memory; C parameter
function [mu_t, sigma_t, sigma_t_norm] = WindEstimator(I_r_IB_hat, B_v_IB_tilde_hat, I_v_IB_hat, C_BI_hat, R, Q, heights, wind_profile_hat, C)
    h = -I_r_IB_hat(3);
    global w_bar_hat
    w_bar_hat_k = [interp1(heights, wind_profile_hat(1,:), h);
                   interp1(heights, wind_profile_hat(2,:), h);
                   0];
    u = w_bar_hat_k - w_bar_hat;
    w_bar_hat = w_bar_hat_k; % store for next timestep
    z = C_BI_hat*I_v_IB_hat - B_v_IB_tilde_hat;
    H = C_BI_hat;

    % Kalman Filter
    global mu
    global sigma

    mu_p = mu + u;
    Sp = sigma + Q;
    sigma = (Sp^-1 + H'/R*H)^-1;
    mu = mu_p + sigma*H'/R*(z-H*mu_p);

    mu_t = mu;
    sigma_t = sigma;
    sigma_t_norm = norm(sigma_t,1);

    % Wind Forcast Error
    global wind_err;

    % data format: [h; ew;];
    % data pushback
    wind_err = [wind_err(:,2:end), [h;
                                    mu_t - w_bar_hat_k]];

end

== matlab function main_simulator/Wind Generator1/MATLAB Function1 ==
  data: V output; V_b input
function V = two_norm(V_b)

    V = norm(V_b);

end

== matlab function main_simulator/MATLAB Function3 ==
  data: B_v_IB_tilde input; I_r_IB input; C_BI input; B_w_IB input; m parameter; g parameter; C_BP parameter; ref_area parameter; S_pd parameter; R parameter; aeroF_est_switch data_store_memory; aeroF_co_sigma data_store_memory; aeroF_co_mu data_store_memory; aeroF_est_ab data_store_memory; C_BW parameter; mu1 output; mu2 output; mu3 output
function [mu1, mu2, mu3] = SteadyGlidingForceCoffMeasure(B_v_IB_tilde,I_r_IB, C_BI, B_w_IB, m, g, C_BP, ref_area, S_pd, R, C_BW)
    
    global aeroF_est_switch;
    global aeroF_co_mu;
    global aeroF_co_sigma;

%     global aeroF_est_ab;
    mu1 = aeroF_co_mu(:,1);
    mu2 = aeroF_co_mu(:,2);
    mu3 = aeroF_co_mu(:,3);
    l = aeroF_est_switch(1);

    if aeroF_est_switch(1) == 0 
        if aeroF_est_switch(2) < 20
            aeroF_est_switch(2) = aeroF_est_switch(2) +1;
        else
            aeroF_est_switch(1) = 1;
        end
        return
    end

        

    if norm(B_w_IB,inf) > 0.08 || aeroF_est_switch(1) == 4
        return
    end


    C_IB = C_BI';
    rpy = [atan2(C_IB(3,2), C_IB(3,3));
          atan2(-C_IB(3,1), sqrt(C_IB(3,2)^2 + C_IB(3,3)^2));
          atan2(C_IB(2,1), C_IB(1,1))];
    
    h = - I_r_IB(3);
    rho = 1.225*(1 - h*2.256e-5)^4.2559;

    P_v_IP_tilde = C_BP\(B_v_IB_tilde);
    u = P_v_IP_tilde(1);
    v = P_v_IP_tilde(2);
    w = P_v_IP_tilde(3);
    alpha = atan(w/u); % angle of attack
    Va = sqrt(u^2+v^2+w^2);
    beta = asin(v/Va); % angle of sideslip
    C_PF = [cos(alpha)*cos(beta), -cos(alpha)*sin(beta), -sin(alpha);
            sin(beta), cos(beta), 0;
            sin(alpha)*cos(beta), -sin(alpha)*sin(beta), cos(alpha)];
    
    % z
    B_F_w = m*g*[-sin(rpy(2));
                sin(rpy(1))*cos(rpy(2));
                cos(rpy(1))*cos(rpy(2))];
    z = 2/rho*B_F_w;

    % H
    W_v_IW_tilde = C_BW\(B_v_IB_tilde);
    H = [ref_area*Va^2*C_BP*C_PF, S_pd*norm(W_v_IW_tilde)*C_BW*W_v_IW_tilde]; %3*4
    

    K = aeroF_co_sigma(:, (4*l-3):(4*l)) * H'/ (H * aeroF_co_sigma(:, (4*l-3):(4*l))*H' + R);
    aeroF_co_mu(:,l) = aeroF_co_mu(:,l) + K * (z - H*aeroF_co_mu(:,l));
    aeroF_co_sigma(:, (4*l-3):(4*l)) = (eye(4) - K*H) * aeroF_co_sigma(:, (4*l-3):(4*l)) * (eye(4) - K*H)' + K*R*K';
    
    aeroF_est_switch(2) = aeroF_est_switch(2) + 1;
    
    if aeroF_est_switch(2) > 60
        aeroF_est_switch(2) = 0;
        aeroF_est_switch(1) = aeroF_est_switch(1) + 1;
    end

end

== matlab function main_simulator/GuidancePDcontroller ==
  data: B_w_IB input; C_BI input; I_r_IB input; e_psi output; delta_l data_store_memory; delta_r data_store_memory; guidance data_store_memory; e_x output; e_y output; GuidanceService data_store_memory; colornum data_store_memory
function [e_psi, e_x, e_y]  = GuidancePDcontroller(B_w_IB, C_BI, I_r_IB)
    global delta_l
    global delta_r
    global guidance
    global GuidanceService
    global colornum
    
    % choose control method
    ctrlmsd = 1; % 0 - psi PD control; 1 - x+y+psi PD control
    
    % get current state
    h = -I_r_IB(3);
    C_IB = C_BI';
    x_now = I_r_IB(1);
    y_now = I_r_IB(2);
    psi_now = atan2(C_IB(2,1), C_IB(1,1));
    
    % plot current state
    hold on;
    colorcode = {"g","b", "c", "m", "#0072BD", "#D95319", "#EDB120", "#7E2F8E", "#77AC30", "#4DBEEE", "#A2142F"};
    states_now = [y_now,                x_now,                h;
                  y_now+1*sin(psi_now), x_now+1*cos(psi_now), h];
    plot3(states_now(:,1), states_now(:,2), states_now(:,3), 'color', colorcode{colornum});

    % default output
    e_psi = 0;
    e_x = 0;
    e_y = 0;

    if isnan(x_now) || isnan(y_now) || isnan(h) || isnan(psi_now)
        disp("Warning: GuidancePDcontroller early return because of NaN value")
        return
    elseif h < 1e-6
        disp("Warning: GuidancePDcontroller early return because h < 1e-6")
        return
    end

    % get guidance
    zero_cnt = sum(guidance==0, 'all');

    if zero_cnt<3 % if guidance received
        x_des = interp1(guidance(3,:), guidance(1,:), h, 'linear','extrap'); 
        y_des = interp1(guidance(3,:), guidance(2,:), h, 'linear','extrap'); 
        psi_des = interp1(guidance(3,:), guidance(4,:), h, 'linear','extrap'); 
        % because of sensor noise, h can be out of bound! 
        % If not extrap, NaN comes which will cause error!

        % plot desired trajectory
        traj = [y_des,                x_des,                h;
                y_des+1*sin(psi_des), x_des+1*cos(psi_des), h];
        plot3(traj(:,1), traj(:,2), traj(:,3), 'r');

        e1 = x_now - x_des;
        e2 = y_now - y_des;

%         if norm([e1, e2]) > 30
%             GuidanceService = 1; % call guidance service again
%             return
%         end

        % PD control
        psi_dot_now = B_w_IB(3); % approximately
        if ctrlmsd == 0
            kp = 3; % kp >= 0
            kd = 0.1; % kd >= 0
            e_psi = warpToPi(psi_now - psi_des); % in [-pi, pi]
            u = kp * e_psi + kd * psi_dot_now;
            delta_l = 0.5 + u; % if u>0, turn left
            delta_r = 0.5 - u;

        elseif ctrlmsd == 1
            kp = 3; % kp >= 0
            kd = 0.1; % kd >= 0
            kpy = 0.02; % kpy >= 0
            kpx = 0.5; % kpx >= 0

            e_x = e1*cos(psi_des) + e2*sin(psi_des);
            e_y = - e1*sin(psi_des) + e2*cos(psi_des);

            psi_des = psi_des - kpy * e_y; % compensate y deviation
            e_psi = warpToPi(psi_now - psi_des); % in [-pi, pi]
            u = kp * e_psi + kd * psi_dot_now;
            ux = kpx * e_x; % compensate x deviation
            
            % heuristic allocation
            u = max(min(u, 0.5),-0.5); % track psi first
            if u > 0
                ux = max(min(ux, 0.5-u), u-0.5); % change delta_s to control velocity
            else
                ux = max(min(ux, 0.5+u), -u-0.5);
            end

            delta_l = 0.5 + u + ux; % if u>0, turn left
            delta_r = 0.5 - u + ux; % if ux>0, slow down
        else
            disp("Warning: control method is not selected!")
        end
    end
end

function alpha = warpToPi(theta)
    theta = mod(theta, 2*pi);
    if theta > pi
        alpha = theta - 2*pi;
    else
        alpha = theta;
    end
end

== matlab function main_simulator/WindPredictViz ==
  data: wind_predict input; viz output; I_r_IB input
function viz = WindPredictViz(wind_predict, I_r_IB)
    viz = [0, 0, 0];
    zero_cnt = sum(wind_predict==0);
    if zero_cnt < 2
        h = -I_r_IB(3);
        mu_x = interp1(wind_predict(1,:), wind_predict(2,:), h);
        mu_y = interp1(wind_predict(1,:), wind_predict(3,:), h);
        mu_z = interp1(wind_predict(1,:), wind_predict(4,:), h);
        viz = [mu_x, mu_y, mu_z];
    end
end

== matlab function main_simulator/MATLAB Function7 ==
  data: u input; y output
function y = motor(u)
    if u>1
        y = 1;
    elseif u<0
        y = 0;
    else
        y = u;
    end
end

== matlab function main_simulator/Aero force and drag ==
  data: airspeed_data output; alpha_deg output; beta_deg output; delta_l input; delta_r input; rho input; B_v_IB_tilde input; P_v_IP_tilde input; B_w_IB input; B_F output; B_M output; cL parameter; cD parameter; b parameter; c parameter; C_BP parameter; ref_area parameter; cM parameter; B_r_BP parameter; c_Dpd parameter; S_pd parameter; B_r_BW parameter; C_BW parameter; cYb parameter
function [airspeed_data, alpha_deg, beta_deg, B_F, B_M] = AeroFM(delta_l, delta_r, rho, B_v_IB_tilde, P_v_IP_tilde, B_w_IB, cL, cD, b, c, C_BP, ref_area, cM, B_r_BP, c_Dpd, S_pd, B_r_BW, C_BW, cYb)
    % control inputs transfer
    delta_s = (delta_l + delta_r) / 2;
    delta_a = delta_r - delta_l;
    
    % B_v_IB_tilde
    u_B = B_v_IB_tilde(1);
    v_B = B_v_IB_tilde(2);
    w_B = B_v_IB_tilde(3);
    V_b = norm(B_v_IB_tilde);
    alpha_B = atan(w_B/u_B);
    beta_B = asin(v_B/V_b);
    airspeed_data = [alpha_B, beta_B, V_b];

    % P_v_IP_tilde = [u, v, w]
    u = P_v_IP_tilde(1);
    v = P_v_IP_tilde(2);
    w = P_v_IP_tilde(3);
    alpha = atan(w/u); % angle of attack
    alpha_deg = alpha / pi * 180;
    Va = sqrt(u^2+v^2+w^2);
    beta = asin(v/Va); % angle of sideslip
    beta_deg = beta / pi * 180;
    C_PF = [cos(alpha)*cos(beta), -cos(alpha)*sin(beta), -sin(alpha);
            sin(beta), cos(beta), 0;
            sin(alpha)*cos(beta), -sin(alpha)*sin(beta), cos(alpha)];

    % P_w_IP = [p, q, r]
    P_w_IP_skew = C_BP\skew(B_w_IB)*C_BP;
    p = P_w_IP_skew(3,2);
    q = P_w_IP_skew(1,3);
    r = P_w_IP_skew(2,1);

    % aero force on parafoil
    P_F_A = C_PF * 0.5 * rho * ref_area * Va^2 * [ - [1, alpha^2, delta_s] * cD;
                                                   - beta * cYb;
                                                   - [1, alpha, delta_s] * cL ];

    % aero moment on parafoil
    c_l = [(b/2/Va)*p, delta_a] * cM(1:2);
    c_m = [1, alpha, (c/2/Va)*q] * cM(3:5);
    c_n = [(b/2/Va)*r, delta_a] * cM(6:7);
    P_M_A = 0.5 * rho * ref_area * Va^2 * [b*c_l; c*c_m; b*c_n];
    

    % aero force on payload
    W_v_IW_tilde = C_BW\(B_v_IB_tilde + cross(B_w_IB, B_r_BW));
    W_F_pd = -0.5*rho*S_pd*c_Dpd*norm(W_v_IW_tilde)*W_v_IW_tilde;

    % total force and moments in body frame
    B_F = C_BP * P_F_A + C_BW * W_F_pd;
    B_M = C_BP * P_M_A + cross(B_r_BP, P_F_A) + cross(B_r_BW, W_F_pd);

%     aeroCofs = [[1, alpha^2, delta_s] * cD, beta * cYb, [1, alpha, delta_s] * cL, c_Dpd];
end

function S = skew(v)
    S = [0,     -v(3),  v(2);
         v(3),  0,      -v(1);
         -v(2), v(1),   0];
end

== matlab function main_simulator/apparent mass ==
  data: B_w_IB input; B_w_IB_dot input; P_v_IP_tilde input; B_F_am output; P_v_IP_tilde_dot input; rho input; B_M_am output; Im parameter; Ii parameter; B_r_BP parameter; C_BP parameter
function [B_F_am, B_M_am] = ApparentMassEffect(B_w_IB, B_w_IB_dot, P_v_IP_tilde, P_v_IP_tilde_dot, rho, Im, Ii, B_r_BP, C_BP)
    
    Iam = rho * Im;
    Iai = rho * Ii;

    % P_w_IP
    P_w_IP_skew = C_BP\skew(B_w_IB)*C_BP;
    P_w_IP = [P_w_IP_skew(3,2);
              P_w_IP_skew(1,3);
              P_w_IP_skew(2,1)];
    
    % P_w_IP_dot
    P_w_IP_dot_skew = C_BP\skew(B_w_IB_dot)*C_BP;
    P_w_IP_dot = [P_w_IP_dot_skew(3,2);
                  P_w_IP_dot_skew(1,3);
                  P_w_IP_dot_skew(2,1)];

    % compute apparent mass effect in parafoil frame
    P_F_am = -(Iam * P_v_IP_tilde_dot + cross(P_w_IP, Iam*P_v_IP_tilde));
    P_M_am = -(Iai * P_w_IP_dot + cross(P_w_IP, Iai*P_w_IP) + cross(P_v_IP_tilde, Iam* P_v_IP_tilde));
    
    % transform
    B_F_am = C_BP * P_F_am;
    B_M_am = C_BP * P_M_am + cross(B_r_BP, P_F_am);

end

function S = skew(v)
    S = [0,     -v(3),  v(2);
         v(3),  0,      -v(1);
         -v(2), v(1),   0];
end

== matlab function main_simulator/Wind Generator/DeltaWindDyn ==
  settings: updateMethod=DISCRETE
  data: delta_w_t input; delta_w_t_dot output; a_w parameter; diag_sigma_zeta parameter
function delta_w_t_dot = DeltaWindDyn(delta_w_t, a_w, diag_sigma_zeta)
    zeta = [sqrt(diag_sigma_zeta(1))*randn();
            sqrt(diag_sigma_zeta(2))*randn();
            sqrt(diag_sigma_zeta(3))*randn()];
    delta_w_t_dot = a_w * delta_w_t + zeta;

end

== matlab function main_simulator/Velovity Transfer ==
  data: B_v_IB_tilde input; B_w_IB input; P_v_IP_tilde output; B_r_BP parameter; C_BP parameter
function P_v_IP_tilde = VelTrans(B_v_IB_tilde, B_w_IB, B_r_BP, C_BP)
    P_v_IP_tilde = C_BP\(B_v_IB_tilde + cross(B_w_IB, B_r_BP));
end
